simulink model "Linear_model"  (R2021b)
settings: Solver=FixedStepAuto  StartTime=0.0  StopTime=30  FixedStep=0.001  RelTol=1e-3  EnableMultiTasking=on
undefined symbols (not defined in the file): F, F_j, F_js, F_s, T_i, T_is, T_ji, T_jis, T_js, T_s
settings Model: Creator=Administrator  LastModifiedBy=Administrator

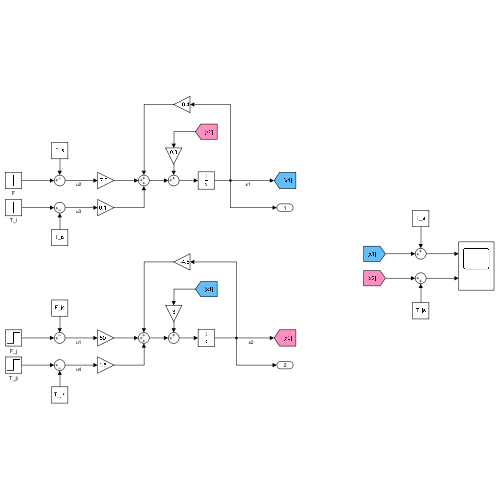
[thumbnail: Simulink's stored preview of the top-level diagram]
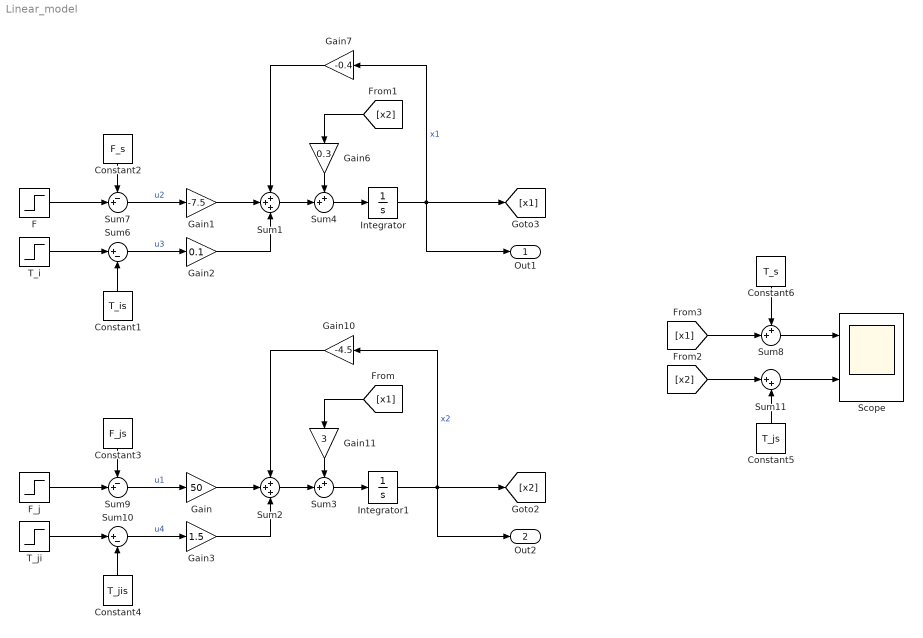
== system Linear_model ==
  Constant1 : Constant  Value=T_is
  Constant2 : Constant  Value=F_s
  Constant3 : Constant  Value=F_js
  Constant4 : Constant  Value=T_jis
  Constant5 : Constant  Value=T_js
  Constant6 : Constant  Value=T_s
  F : Step  Time=0  After=F  SampleTime=0
  F_j : Step  Time=0  After=F_j  SampleTime=0
  Gain : Gain  Gain=50
  Gain1 : Gain  Gain=-7.5
  Gain10 : Gain  Gain=-4.5
  Gain11 : Gain  Gain=3
  Gain2 : Gain  Gain=0.1
  Gain3 : Gain  Gain=1.5
  Gain6 : Gain  Gain=0.3
  Gain7 : Gain  Gain=-0.4
  Integrator : Integrator
  Integrator1 : Integrator
  Scope : Scope  NumInputPorts=2
  Sum1 : Sum  Inputs=+++
  Sum10 : Sum  Inputs=|+-
  Sum11 : Sum  Inputs=|++
  Sum2 : Sum  Inputs=+++
  Sum3 : Sum  Inputs=++|
  Sum4 : Sum  Inputs=++|
  Sum6 : Sum  Inputs=|+-
  Sum7 : Sum  Inputs=-+|
  Sum8 : Sum  Inputs=++|
  Sum9 : Sum  Inputs=-+|
  T_i : Step  Time=0  After=T_i  SampleTime=0
  T_ji : Step  Time=0  After=T_ji  SampleTime=0
  Out1 : Outport
  Out2 : Outport  Port=2
  wires:
  [x1] -> Sum8/2
  Sum8/1 -> Scope/1
  Sum11/1 -> Scope/2
  [x2] -> Sum11/1
  Constant5/1 -> Sum11/2
  Constant6/1 -> Sum8/1
  F/1 -> Sum7/2
  Gain/1 -> Sum2/2
  F_j/1 -> Sum9/2
  Integrator/1 -> Out1/1, [x1], Gain7/1  "x1"
  Sum10/1 -> Gain3/1  "u4"
  Sum6/1 -> Gain2/1  "u3"
  Gain11/1 -> Sum3/1
  Sum9/1 -> Gain/1  "u1"
  [x2] -> Gain6/1
  Sum1/1 -> Sum4/2
  Gain7/1 -> Sum1/1
  Sum7/1 -> Gain1/1  "u2"
  Gain10/1 -> Sum2/1
  Sum4/1 -> Integrator/1
  T_i/1 -> Sum6/1
  [x1] -> Gain11/1
  Gain3/1 -> Sum2/3
  Integrator1/1 -> Out2/1, Gain10/1, [x2]  "x2"
  Gain1/1 -> Sum1/2
  Constant2/1 -> Sum7/1
  Sum2/1 -> Sum3/2
  Constant1/1 -> Sum6/2
  Gain6/1 -> Sum4/1
  Sum3/1 -> Integrator1/1
  T_ji/1 -> Sum10/1
  Gain2/1 -> Sum1/3
  Constant3/1 -> Sum9/1
  Constant4/1 -> Sum10/2
